simulink model "state_space_all2"  (R2018a)
settings: Solver=FixedStepAuto  StartTime=0.0  StopTime=3  FixedStep=tm  MaxStep=1e-4  RelTol=1e-5  AbsTol=1e-5
InitFcn:
  | SimulinkInit_linea_transmision
values from neighbouring files (symbols this model uses):
  b = 4.91    [SimulinkInit_linea_transmision.m]
  C = 1    [SimulinkInit_linea_transmision.m]
  C1 = 22e-6    (= 2.2e-05)    [SimulinkInit_linea_transmision.m]
  C2 = 22e-6    (= 2.2e-05)    [SimulinkInit_linea_transmision.m]
  C3 = 610e-6    (= 0.00061)    [SimulinkInit_linea_transmision.m]
  Cl = 20000e-6    (= 0.02)    [SimulinkInit_linea_transmision.m]
  Jd = 0.3    [SimulinkInit_linea_transmision.m]
  K = 25    [SimulinkInit_linea_transmision.m]    (also in uio_linear.m = K1+E*H)
  K1 = 9.66    [SimulinkInit_linea_transmision.m]    (also in uio_linear.m = K1')
  K11 = 0.8    [SimulinkInit_linea_transmision.m]
  K1d = 1.15    [SimulinkInit_linea_transmision.m]
  K2 = 6.97    [SimulinkInit_linea_transmision.m]
  K22 = 0.2    [SimulinkInit_linea_transmision.m]
  K2d = 1    [SimulinkInit_linea_transmision.m]
  K3 = 31.8    [SimulinkInit_linea_transmision.m]
  K33 = 0.23    [SimulinkInit_linea_transmision.m]
  K3d = 1    [SimulinkInit_linea_transmision.m]
  K4 = 15.1    [SimulinkInit_linea_transmision.m]
  Kd = 0.02    [SimulinkInit_linea_transmision.m]
  Kdc = 0.02    [SimulinkInit_linea_transmision.m]
  Kf = 1    [SimulinkInit_linea_transmision.m]
  Kh = 1.2    [SimulinkInit_linea_transmision.m]
  Ks = 21.5    [SimulinkInit_linea_transmision.m]
  Ksc = 3    [SimulinkInit_linea_transmision.m]
  Kv = 1    [SimulinkInit_linea_transmision.m]
  L = 5.2    [SimulinkInit_linea_transmision.m]
  L1 = 40e-3    (= 0.04)    [SimulinkInit_linea_transmision.m]
  L2 = 30e-3    (= 0.03)    [SimulinkInit_linea_transmision.m]
  L3 = 5e-3    (= 0.005)    [SimulinkInit_linea_transmision.m]
  L4 = 35e-6    (= 3.5e-05)    [SimulinkInit_linea_transmision.m]
  L5 = 22e-6    (= 2.2e-05)    [SimulinkInit_linea_transmision.m]
  L6 = 10e-6    (= 1e-05)    [SimulinkInit_linea_transmision.m]
  Pd = 0.1    [SimulinkInit_linea_transmision.m]
  R = 10    [SimulinkInit_linea_transmision.m]
  R1 = 0.1    [SimulinkInit_linea_transmision.m]
  R2 = 0.2    [SimulinkInit_linea_transmision.m]
  R3 = 1e-3    (= 0.001)    [SimulinkInit_linea_transmision.m]
  R4 = 0.005    [SimulinkInit_linea_transmision.m]
  R5 = 0.0012    [SimulinkInit_linea_transmision.m]
  R6 = 0.001    [SimulinkInit_linea_transmision.m]
  RL = 10    [SimulinkInit_linea_transmision.m]
  Sbin = 13.8    [SimulinkInit_linea_transmision.m]
  Svin = 2.91    [SimulinkInit_linea_transmision.m]
  T1 = 0.4    [SimulinkInit_linea_transmision.m]
  T2 = 1    [SimulinkInit_linea_transmision.m]
  T3 = 15    [SimulinkInit_linea_transmision.m]
  T4 = 2.5    [SimulinkInit_linea_transmision.m]
  Tao1d = 0.5    [SimulinkInit_linea_transmision.m]
  Tao2d = 0.125    [SimulinkInit_linea_transmision.m]
  Tcd = 0.2    [SimulinkInit_linea_transmision.m]
  Tcr = 0.01    [SimulinkInit_linea_transmision.m]
  Tf = 0.04    [SimulinkInit_linea_transmision.m]
  Tr = 950    [SimulinkInit_linea_transmision.m]
  Tt = 450    [SimulinkInit_linea_transmision.m]
  Ttd = 0.04    [SimulinkInit_linea_transmision.m]
  Tv = 0.05    [SimulinkInit_linea_transmision.m]
  V = 20    [SimulinkInit_linea_transmision.m]
  wref = 70000    [SimulinkInit_linea_transmision.m]
  X_acid = 1.2    [SimulinkInit_linea_transmision.m]
  X_meth = 0.35    [SimulinkInit_linea_transmision.m]
  Z = 3    [SimulinkInit_linea_transmision.m]
undefined symbols (not defined in the file or in its folder): Ad, ataque, Bd, c11, c12, c13, c14, C1o, c21, c22, c23, c24, C2o, c31, c32, c33, c34, C3o, c41, c42, c43, c44, C4o, Cd, F1, F2, F3, F4, H1, H2, H3, H4, K1U, K2U, K3U, K4U, T1s, T2s, T3s, T4s, T5s, tao1, tao2, taod, tm
libraries: neural x277, dsparch4 x4, powerlib_meascontrol x4, mpclib x1, simulink x1
(part 2 of 15)

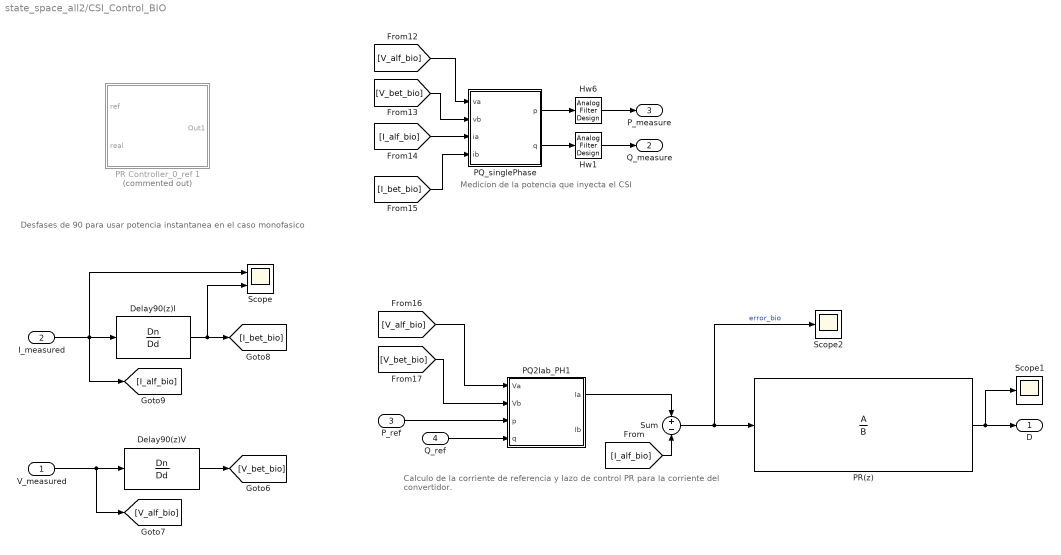
== system state_space_all2/CSI_Control_BIO ==
  note: Medicion de la potencia que inyecta el CSI
  note: Desfases de 90 para usar potencia
      | instantanea en el caso monofasico
  note: Calculo de la corriente de referencia
      | y lazo de control PR para la corriente
      | del convertidor.
  V_measured : Inport
  I_measured : Inport  Port=2
  P_ref : Inport  Port=3
  Q_ref : Inport  Port=4
  Delay90(z)I : DiscreteTransferFcn  Numerator=Dn  Denominator=Dd  SampleTime=T
  Delay90(z)V : DiscreteTransferFcn  Numerator=Dn  Denominator=Dd  SampleTime=T
  Hw1 : dsparch4/Analog Filter Design  method=Bessel  filttype=Lowpass  N=4  Wlo=30*2*pi  Whi=80  Rp=2  Rs=80
  Hw6 : dsparch4/Analog Filter Design  method=Bessel  filttype=Lowpass  N=4  Wlo=30*2*pi  Whi=80  Rp=2  Rs=80
  PQ2Iab_PH1 : MATLAB Function  TreatAsAtomicUnit=on
  PQ_singlePhase : MATLAB Function  TreatAsAtomicUnit=on
  PR Controller_0_ref 1 : Subsystem  Commented=on  mask{Kp=40/100, Ki=200, wa=2, w0=60*2*pi, st_time=1e-3}
      mask prompts: Kp "Ganancia Proporcional"; Ki "Ganancia Integral"; wa "Ancho camapana resonancia"; w0 "Frecuencia Central"; st_time "Tiempo muerto (Start)"
      mask Display:
      | port_label('input',1,'ref')
      | port_label('input',2,'sens')
      | port_label('output',1,'out')
      | 
      | plot(.4+[0:.01:pi/10], .32+sin(40*[0:.01:pi/10])/13)
      | 
      | plot([.4 .6],.05+[.5 .7])
      | plot([.4 .6],.05+[.9 .7])
      | plot([.4 .4],.05+[.9 .5])
      | 
      | text(.27,.37,'\fontsize{25} \int', 'texmode', 'on')
  PR(z) : DiscreteTransferFcn  Numerator=A  Denominator=B  SampleTime=T
  Scope : Scope  NumInputPorts=2
  Scope1 : Scope
  Scope2 : Scope
  Sum : Sum  Inputs=+-
  D : Outport
  Q_measure : Outport  Port=2
  P_measure : Outport  Port=3
  wires:
  I_measured/1 -> Scope/1, Delay90(z)I/1, [I_alf_bio]
  [V_bet_bio] -> PQ2Iab_PH1/2(Vb)
  Delay90(z)I/1 -> Scope/2, [I_bet_bio]
  [I_bet_bio] -> PQ_singlePhase/4(ib)
  [I_alf_bio] -> PQ_singlePhase/3(ia)
  [V_alf_bio] -> PQ2Iab_PH1/1(Va)
  Delay90(z)V/1 -> [V_bet_bio]
  [V_bet_bio] -> PQ_singlePhase/2(vb)
  [V_alf_bio] -> PQ_singlePhase/1(va)
  V_measured/1 -> Delay90(z)V/1, [V_alf_bio]
  P_ref/1 -> PQ2Iab_PH1/3(p)
  Q_ref/1 -> PQ2Iab_PH1/4(q)
  Sum/1 -> Scope2/1, PR(z)/1  "error_bio"
  [I_alf_bio] -> Sum/2
  PQ2Iab_PH1/1(Ia) -> Sum/1
  PR(z)/1 -> Scope1/1, D/1
  PQ_singlePhase/2(q) -> Hw1/1
  Hw1/1 -> Q_measure/1
  PQ_singlePhase/1(p) -> Hw6/1
  Hw6/1 -> P_measure/1

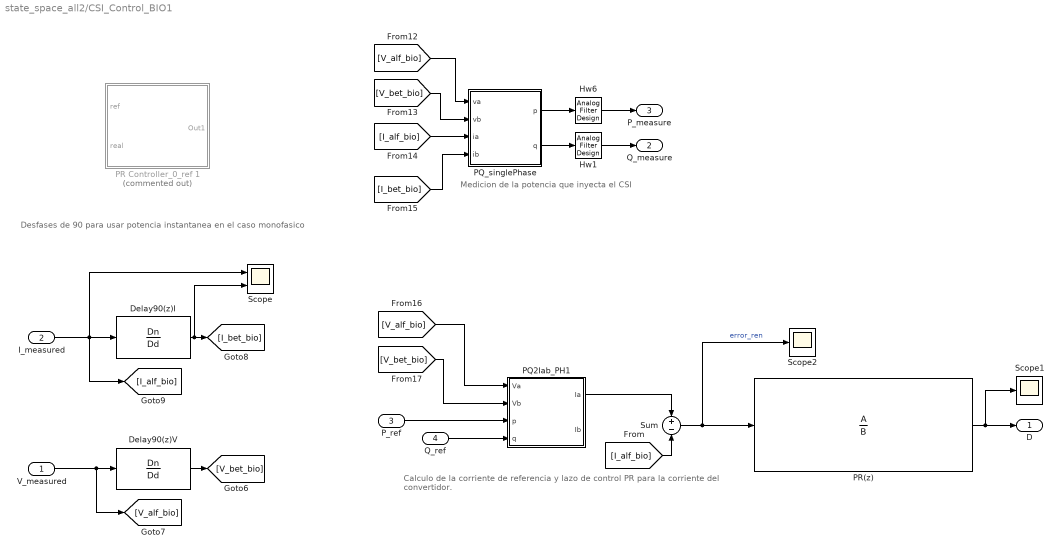
== system state_space_all2/CSI_Control_BIO1 ==
  note: Medicion de la potencia que inyecta el CSI
  note: Desfases de 90 para usar potencia
      | instantanea en el caso monofasico
  note: Calculo de la corriente de referencia
      | y lazo de control PR para la corriente
      | del convertidor.
  V_measured : Inport
  I_measured : Inport  Port=2
  P_ref : Inport  Port=3
  Q_ref : Inport  Port=4
  Delay90(z)I : DiscreteTransferFcn  Numerator=Dn  Denominator=Dd  SampleTime=T
  Delay90(z)V : DiscreteTransferFcn  Numerator=Dn  Denominator=Dd  SampleTime=T
  Hw1 : dsparch4/Analog Filter Design  method=Bessel  filttype=Lowpass  N=4  Wlo=30*2*pi  Whi=80  Rp=2  Rs=80
  Hw6 : dsparch4/Analog Filter Design  method=Bessel  filttype=Lowpass  N=4  Wlo=30*2*pi  Whi=80  Rp=2  Rs=80
  PQ2Iab_PH1 : MATLAB Function  TreatAsAtomicUnit=on
  PQ_singlePhase : MATLAB Function  TreatAsAtomicUnit=on
  PR Controller_0_ref 1 : Subsystem  Commented=on  mask{Kp=40/100, Ki=200, wa=2, w0=60*2*pi, st_time=1e-3}
      mask prompts: Kp "Ganancia Proporcional"; Ki "Ganancia Integral"; wa "Ancho camapana resonancia"; w0 "Frecuencia Central"; st_time "Tiempo muerto (Start)"
      mask Display:
      | port_label('input',1,'ref')
      | port_label('input',2,'sens')
      | port_label('output',1,'out')
      | 
      | plot(.4+[0:.01:pi/10], .32+sin(40*[0:.01:pi/10])/13)
      | 
      | plot([.4 .6],.05+[.5 .7])
      | plot([.4 .6],.05+[.9 .7])
      | plot([.4 .4],.05+[.9 .5])
      | 
      | text(.27,.37,'\fontsize{25} \int', 'texmode', 'on')
  PR(z) : DiscreteTransferFcn  Numerator=A  Denominator=B  SampleTime=T
  Scope : Scope  NumInputPorts=2
  Scope1 : Scope
  Scope2 : Scope
  Sum : Sum  Inputs=+-
  D : Outport
  Q_measure : Outport  Port=2
  P_measure : Outport  Port=3
  wires:
  I_measured/1 -> Scope/1, Delay90(z)I/1, [I_alf_bio]
  [V_bet_bio] -> PQ2Iab_PH1/2(Vb)
  Delay90(z)I/1 -> Scope/2, [I_bet_bio]
  [I_bet_bio] -> PQ_singlePhase/4(ib)
  [I_alf_bio] -> PQ_singlePhase/3(ia)
  [V_alf_bio] -> PQ2Iab_PH1/1(Va)
  Delay90(z)V/1 -> [V_bet_bio]
  [V_bet_bio] -> PQ_singlePhase/2(vb)
  [V_alf_bio] -> PQ_singlePhase/1(va)
  V_measured/1 -> Delay90(z)V/1, [V_alf_bio]
  P_ref/1 -> PQ2Iab_PH1/3(p)
  Q_ref/1 -> PQ2Iab_PH1/4(q)
  Sum/1 -> Scope2/1, PR(z)/1  "error_ren"
  [I_alf_bio] -> Sum/2
  PQ2Iab_PH1/1(Ia) -> Sum/1
  PR(z)/1 -> Scope1/1, D/1
  PQ_singlePhase/2(q) -> Hw1/1
  Hw1/1 -> Q_measure/1
  PQ_singlePhase/1(p) -> Hw6/1
  Hw6/1 -> P_measure/1

== system state_space_all2/Control PR VSI1 ==
  Ierror : Inport
  Constant2 : Constant  Value=0
  Gain2 : Gain  Gain=.002
  Sum5 : Sum  Inputs=+|+
  Sum9 : Sum  Inputs=|++
  Transfer Fcn2 : TransferFcn  Numerator=[2 0]  Denominator=[1 2 (2*pi*60)^2]
  d : Outport
  wires:
  Constant2/1 -> Sum9/2
  Sum5/1 -> Sum9/1
  Transfer Fcn2/1 -> Sum5/2
  Gain2/1 -> Sum5/1
  Ierror/1 -> Transfer Fcn2/1, Gain2/1
  Sum9/1 -> d/1

== system state_space_all2/Diesel Generator2 ==
  in : Inport
  Par de Carga : Inport  Port=2
  " 1" : Gain  Gain=K1d
  " Generador1" : Gain  Gain=1/2
  Actuador1 : TransferFcn  Numerator=[K3d*K2d]  Denominator=[Tao2d 1]
  Dinámica en el eje1 : TransferFcn  Numerator=[(Jd*Pd)]  Denominator=[1 (Jd*Pd)]
  Gain1 : Gain  Gain=12000
  Motor de Combustión1 : TransportDelay  DelayTime=Tao1d
  Sum2 : Sum  Inputs=|+-
  Speed : Outport
  Power : Outport  Port=2
  caudal : Outport  Port=3
  wires:
  " 1"/1 -> Motor de Combustión1/1
  " Generador1"/1 -> Gain1/1
  Motor de Combustión1/1 -> Sum2/1
  Actuador1/1 -> caudal/1, " 1"/1
  Dinámica en el eje1/1 -> Speed/1, " Generador1"/1  "Velocidad"
  Sum2/1 -> Dinámica en el eje1/1
  in/1 -> Actuador1/1
  Par de Carga/1 -> Sum2/2
  Gain1/1 -> Power/1

== system state_space_all2/Function Fitting Neural Network ==
  Input : Inport  PortDimensions=47
      mask Display: e = 0.06;c1 = [120 230 180]/255;c2 = ([120 230 180]+0)/(256+128);c3 = ([120 230 180]+128)/(256+128);patch([0 1 1 0],[0 0 1 1],c1);patch([0 1 1 1-e 1-e 0+e],[0 0 1 1-e 0+e 0+e],c2);patch([0 0 1 1-e 0+e 0+e],[0 1 1 1-e 1-e 0+e],c3);plot([0 1 1 0 0],[0 0 1 1 0]);
  Layer 1 : Subsystem
      mask Display: e = 0.06;c1 = [120 150 230]/255;c2 = ([120 150 230]+0)/383;c3 = ([120 150 230]+128)/383;patch([0 1 1 0],[0 0 1 1],c1);patch([0 1 1 1-e 1-e 0+e],[0 0 1 1-e 0+e 0+e],c2);patch([0 0 1 1-e 0+e 0+e],[0 1 1 1-e 1-e 0+e],c3);plot([0 1 1 0 0],[0 0 1 1 0]);
  Layer 2 : Subsystem
      mask Display: e = 0.06;c1 = [120 150 230]/255;c2 = ([120 150 230]+0)/383;c3 = ([120 150 230]+128)/383;patch([0 1 1 0],[0 0 1 1],c1);patch([0 1 1 1-e 1-e 0+e],[0 0 1 1-e 0+e 0+e],c2);patch([0 0 1 1-e 0+e 0+e],[0 1 1 1-e 1-e 0+e],c3);plot([0 1 1 0 0],[0 0 1 1 0]);
  Layer 3 : Subsystem
      mask Display: e = 0.06;c1 = [120 150 230]/255;c2 = ([120 150 230]+0)/383;c3 = ([120 150 230]+128)/383;patch([0 1 1 0],[0 0 1 1],c1);patch([0 1 1 1-e 1-e 0+e],[0 0 1 1-e 0+e 0+e],c2);patch([0 0 1 1-e 0+e 0+e],[0 1 1 1-e 1-e 0+e],c3);plot([0 1 1 0 0],[0 0 1 1 0]);
  Process Input 1 : Subsystem
      mask Display: e = 0.06;c1 = [120 150 230]/255;c2 = ([120 150 230]+0)/383;c3 = ([120 150 230]+128)/383;patch([0 1 1 0],[0 0 1 1],c1);patch([0 1 1 1-e 1-e 0+e],[0 0 1 1-e 0+e 0+e],c2);patch([0 0 1 1-e 0+e 0+e],[0 1 1 1-e 1-e 0+e],c3);plot([0 1 1 0 0],[0 0 1 1 0]);
  Process Output 1 : Subsystem
      mask Display: e = 0.06;c1 = [120 150 230]/255;c2 = ([120 150 230]+0)/383;c3 = ([120 150 230]+128)/383;patch([0 1 1 0],[0 0 1 1],c1);patch([0 1 1 1-e 1-e 0+e],[0 0 1 1-e 0+e 0+e],c2);patch([0 0 1 1-e 0+e 0+e],[0 1 1 1-e 1-e 0+e],c3);plot([0 1 1 0 0],[0 0 1 1 0]);
  Output : Outport  InitialOutput=[0;0;0;0]
      mask Display: e = 0.06;c1 = [120 230 180]/255;c2 = ([120 230 180]+0)/(256+128);c3 = ([120 230 180]+128)/(256+128);patch([0 1 1 0],[0 0 1 1],c1);patch([0 1 1 1-e 1-e 0+e],[0 0 1 1-e 0+e 0+e],c2);patch([0 0 1 1-e 0+e 0+e],[0 1 1 1-e 1-e 0+e],c3);plot([0 1 1 0 0],[0 0 1 1 0]);
  wires:
  Input/1 -> Process Input 1/1(x)
  Process Output 1/1(y) -> Output/1
  Process Input 1/1(p) -> Layer 1/1("p{1}")
  Layer 1/1("a{1}") -> [feedback1]
  [feedback1] -> Layer 2/1("a{1} ")
  Layer 2/1("a{2}") -> [feedback2]
  [feedback2] -> Layer 3/1("a{2} ")
  Layer 3/1("a{3}") -> Process Output 1/1(a)

== system state_space_all2/Function Fitting Neural Network1 ==
  Input : Inport  PortDimensions=44  SampleTime=4e-05
      mask Display: e = 0.06;c1 = [120 230 180]/255;c2 = ([120 230 180]+0)/(256+128);c3 = ([120 230 180]+128)/(256+128);patch([0 1 1 0],[0 0 1 1],c1);patch([0 1 1 1-e 1-e 0+e],[0 0 1 1-e 0+e 0+e],c2);patch([0 0 1 1-e 0+e 0+e],[0 1 1 1-e 1-e 0+e],c3);plot([0 1 1 0 0],[0 0 1 1 0]);
  Layer 1 : Subsystem
      mask Display: e = 0.06;c1 = [120 150 230]/255;c2 = ([120 150 230]+0)/383;c3 = ([120 150 230]+128)/383;patch([0 1 1 0],[0 0 1 1],c1);patch([0 1 1 1-e 1-e 0+e],[0 0 1 1-e 0+e 0+e],c2);patch([0 0 1 1-e 0+e 0+e],[0 1 1 1-e 1-e 0+e],c3);plot([0 1 1 0 0],[0 0 1 1 0]);
  Layer 2 : Subsystem
      mask Display: e = 0.06;c1 = [120 150 230]/255;c2 = ([120 150 230]+0)/383;c3 = ([120 150 230]+128)/383;patch([0 1 1 0],[0 0 1 1],c1);patch([0 1 1 1-e 1-e 0+e],[0 0 1 1-e 0+e 0+e],c2);patch([0 0 1 1-e 0+e 0+e],[0 1 1 1-e 1-e 0+e],c3);plot([0 1 1 0 0],[0 0 1 1 0]);
  Layer 3 : Subsystem
      mask Display: e = 0.06;c1 = [120 150 230]/255;c2 = ([120 150 230]+0)/383;c3 = ([120 150 230]+128)/383;patch([0 1 1 0],[0 0 1 1],c1);patch([0 1 1 1-e 1-e 0+e],[0 0 1 1-e 0+e 0+e],c2);patch([0 0 1 1-e 0+e 0+e],[0 1 1 1-e 1-e 0+e],c3);plot([0 1 1 0 0],[0 0 1 1 0]);
  Layer 4 : Subsystem
      mask Display: e = 0.06;c1 = [120 150 230]/255;c2 = ([120 150 230]+0)/383;c3 = ([120 150 230]+128)/383;patch([0 1 1 0],[0 0 1 1],c1);patch([0 1 1 1-e 1-e 0+e],[0 0 1 1-e 0+e 0+e],c2);patch([0 0 1 1-e 0+e 0+e],[0 1 1 1-e 1-e 0+e],c3);plot([0 1 1 0 0],[0 0 1 1 0]);
  Process Input 1 : Subsystem
      mask Display: e = 0.06;c1 = [120 150 230]/255;c2 = ([120 150 230]+0)/383;c3 = ([120 150 230]+128)/383;patch([0 1 1 0],[0 0 1 1],c1);patch([0 1 1 1-e 1-e 0+e],[0 0 1 1-e 0+e 0+e],c2);patch([0 0 1 1-e 0+e 0+e],[0 1 1 1-e 1-e 0+e],c3);plot([0 1 1 0 0],[0 0 1 1 0]);
  Process Output 1 : Subsystem
      mask Display: e = 0.06;c1 = [120 150 230]/255;c2 = ([120 150 230]+0)/383;c3 = ([120 150 230]+128)/383;patch([0 1 1 0],[0 0 1 1],c1);patch([0 1 1 1-e 1-e 0+e],[0 0 1 1-e 0+e 0+e],c2);patch([0 0 1 1-e 0+e 0+e],[0 1 1 1-e 1-e 0+e],c3);plot([0 1 1 0 0],[0 0 1 1 0]);
  Output : Outport  InitialOutput=0
      mask Display: e = 0.06;c1 = [120 230 180]/255;c2 = ([120 230 180]+0)/(256+128);c3 = ([120 230 180]+128)/(256+128);patch([0 1 1 0],[0 0 1 1],c1);patch([0 1 1 1-e 1-e 0+e],[0 0 1 1-e 0+e 0+e],c2);patch([0 0 1 1-e 0+e 0+e],[0 1 1 1-e 1-e 0+e],c3);plot([0 1 1 0 0],[0 0 1 1 0]);
  wires:
  Input/1 -> Process Input 1/1(x)
  Process Output 1/1(y) -> Output/1
  Process Input 1/1(p) -> Layer 1/1("p{1}")
  Layer 1/1("a{1}") -> [feedback1]
  [feedback1] -> Layer 2/1("a{1} ")
  Layer 2/1("a{2}") -> [feedback2]
  [feedback2] -> Layer 3/1("a{2} ")
  Layer 3/1("a{3}") -> [feedback3]
  [feedback3] -> Layer 4/1("a{3} ")
  Layer 4/1("a{4}") -> Process Output 1/1(a)

== system state_space_all2/Function Fitting Neural Network2 ==
  Input : Inport  PortDimensions=44  SampleTime=4e-05
      mask Display: e = 0.06;c1 = [120 230 180]/255;c2 = ([120 230 180]+0)/(256+128);c3 = ([120 230 180]+128)/(256+128);patch([0 1 1 0],[0 0 1 1],c1);patch([0 1 1 1-e 1-e 0+e],[0 0 1 1-e 0+e 0+e],c2);patch([0 0 1 1-e 0+e 0+e],[0 1 1 1-e 1-e 0+e],c3);plot([0 1 1 0 0],[0 0 1 1 0]);
  Layer 1 : Subsystem
      mask Display: e = 0.06;c1 = [120 150 230]/255;c2 = ([120 150 230]+0)/383;c3 = ([120 150 230]+128)/383;patch([0 1 1 0],[0 0 1 1],c1);patch([0 1 1 1-e 1-e 0+e],[0 0 1 1-e 0+e 0+e],c2);patch([0 0 1 1-e 0+e 0+e],[0 1 1 1-e 1-e 0+e],c3);plot([0 1 1 0 0],[0 0 1 1 0]);
  Layer 2 : Subsystem
      mask Display: e = 0.06;c1 = [120 150 230]/255;c2 = ([120 150 230]+0)/383;c3 = ([120 150 230]+128)/383;patch([0 1 1 0],[0 0 1 1],c1);patch([0 1 1 1-e 1-e 0+e],[0 0 1 1-e 0+e 0+e],c2);patch([0 0 1 1-e 0+e 0+e],[0 1 1 1-e 1-e 0+e],c3);plot([0 1 1 0 0],[0 0 1 1 0]);
  Layer 3 : Subsystem
      mask Display: e = 0.06;c1 = [120 150 230]/255;c2 = ([120 150 230]+0)/383;c3 = ([120 150 230]+128)/383;patch([0 1 1 0],[0 0 1 1],c1);patch([0 1 1 1-e 1-e 0+e],[0 0 1 1-e 0+e 0+e],c2);patch([0 0 1 1-e 0+e 0+e],[0 1 1 1-e 1-e 0+e],c3);plot([0 1 1 0 0],[0 0 1 1 0]);
  Layer 4 : Subsystem
      mask Display: e = 0.06;c1 = [120 150 230]/255;c2 = ([120 150 230]+0)/383;c3 = ([120 150 230]+128)/383;patch([0 1 1 0],[0 0 1 1],c1);patch([0 1 1 1-e 1-e 0+e],[0 0 1 1-e 0+e 0+e],c2);patch([0 0 1 1-e 0+e 0+e],[0 1 1 1-e 1-e 0+e],c3);plot([0 1 1 0 0],[0 0 1 1 0]);
  Process Input 1 : Subsystem
      mask Display: e = 0.06;c1 = [120 150 230]/255;c2 = ([120 150 230]+0)/383;c3 = ([120 150 230]+128)/383;patch([0 1 1 0],[0 0 1 1],c1);patch([0 1 1 1-e 1-e 0+e],[0 0 1 1-e 0+e 0+e],c2);patch([0 0 1 1-e 0+e 0+e],[0 1 1 1-e 1-e 0+e],c3);plot([0 1 1 0 0],[0 0 1 1 0]);
  Process Output 1 : Subsystem
      mask Display: e = 0.06;c1 = [120 150 230]/255;c2 = ([120 150 230]+0)/383;c3 = ([120 150 230]+128)/383;patch([0 1 1 0],[0 0 1 1],c1);patch([0 1 1 1-e 1-e 0+e],[0 0 1 1-e 0+e 0+e],c2);patch([0 0 1 1-e 0+e 0+e],[0 1 1 1-e 1-e 0+e],c3);plot([0 1 1 0 0],[0 0 1 1 0]);
  Output : Outport  InitialOutput=0
      mask Display: e = 0.06;c1 = [120 230 180]/255;c2 = ([120 230 180]+0)/(256+128);c3 = ([120 230 180]+128)/(256+128);patch([0 1 1 0],[0 0 1 1],c1);patch([0 1 1 1-e 1-e 0+e],[0 0 1 1-e 0+e 0+e],c2);patch([0 0 1 1-e 0+e 0+e],[0 1 1 1-e 1-e 0+e],c3);plot([0 1 1 0 0],[0 0 1 1 0]);
  wires:
  Input/1 -> Process Input 1/1(x)
  Process Output 1/1(y) -> Output/1
  Process Input 1/1(p) -> Layer 1/1("p{1}")
  Layer 1/1("a{1}") -> [feedback1]
  [feedback1] -> Layer 2/1("a{1} ")
  Layer 2/1("a{2}") -> [feedback2]
  [feedback2] -> Layer 3/1("a{2} ")
  Layer 3/1("a{3}") -> [feedback3]
  [feedback3] -> Layer 4/1("a{3} ")
  Layer 4/1("a{4}") -> Process Output 1/1(a)

== system state_space_all2/Function Fitting Neural Network3 ==
  Input : Inport  PortDimensions=44  SampleTime=4e-05
      mask Display: e = 0.06;c1 = [120 230 180]/255;c2 = ([120 230 180]+0)/(256+128);c3 = ([120 230 180]+128)/(256+128);patch([0 1 1 0],[0 0 1 1],c1);patch([0 1 1 1-e 1-e 0+e],[0 0 1 1-e 0+e 0+e],c2);patch([0 0 1 1-e 0+e 0+e],[0 1 1 1-e 1-e 0+e],c3);plot([0 1 1 0 0],[0 0 1 1 0]);
  Layer 1 : Subsystem
      mask Display: e = 0.06;c1 = [120 150 230]/255;c2 = ([120 150 230]+0)/383;c3 = ([120 150 230]+128)/383;patch([0 1 1 0],[0 0 1 1],c1);patch([0 1 1 1-e 1-e 0+e],[0 0 1 1-e 0+e 0+e],c2);patch([0 0 1 1-e 0+e 0+e],[0 1 1 1-e 1-e 0+e],c3);plot([0 1 1 0 0],[0 0 1 1 0]);
  Layer 2 : Subsystem
      mask Display: e = 0.06;c1 = [120 150 230]/255;c2 = ([120 150 230]+0)/383;c3 = ([120 150 230]+128)/383;patch([0 1 1 0],[0 0 1 1],c1);patch([0 1 1 1-e 1-e 0+e],[0 0 1 1-e 0+e 0+e],c2);patch([0 0 1 1-e 0+e 0+e],[0 1 1 1-e 1-e 0+e],c3);plot([0 1 1 0 0],[0 0 1 1 0]);
  Layer 3 : Subsystem
      mask Display: e = 0.06;c1 = [120 150 230]/255;c2 = ([120 150 230]+0)/383;c3 = ([120 150 230]+128)/383;patch([0 1 1 0],[0 0 1 1],c1);patch([0 1 1 1-e 1-e 0+e],[0 0 1 1-e 0+e 0+e],c2);patch([0 0 1 1-e 0+e 0+e],[0 1 1 1-e 1-e 0+e],c3);plot([0 1 1 0 0],[0 0 1 1 0]);
  Layer 4 : Subsystem
      mask Display: e = 0.06;c1 = [120 150 230]/255;c2 = ([120 150 230]+0)/383;c3 = ([120 150 230]+128)/383;patch([0 1 1 0],[0 0 1 1],c1);patch([0 1 1 1-e 1-e 0+e],[0 0 1 1-e 0+e 0+e],c2);patch([0 0 1 1-e 0+e 0+e],[0 1 1 1-e 1-e 0+e],c3);plot([0 1 1 0 0],[0 0 1 1 0]);
  Process Input 1 : Subsystem
      mask Display: e = 0.06;c1 = [120 150 230]/255;c2 = ([120 150 230]+0)/383;c3 = ([120 150 230]+128)/383;patch([0 1 1 0],[0 0 1 1],c1);patch([0 1 1 1-e 1-e 0+e],[0 0 1 1-e 0+e 0+e],c2);patch([0 0 1 1-e 0+e 0+e],[0 1 1 1-e 1-e 0+e],c3);plot([0 1 1 0 0],[0 0 1 1 0]);
  Process Output 1 : Subsystem
      mask Display: e = 0.06;c1 = [120 150 230]/255;c2 = ([120 150 230]+0)/383;c3 = ([120 150 230]+128)/383;patch([0 1 1 0],[0 0 1 1],c1);patch([0 1 1 1-e 1-e 0+e],[0 0 1 1-e 0+e 0+e],c2);patch([0 0 1 1-e 0+e 0+e],[0 1 1 1-e 1-e 0+e],c3);plot([0 1 1 0 0],[0 0 1 1 0]);
  Output : Outport  InitialOutput=0
      mask Display: e = 0.06;c1 = [120 230 180]/255;c2 = ([120 230 180]+0)/(256+128);c3 = ([120 230 180]+128)/(256+128);patch([0 1 1 0],[0 0 1 1],c1);patch([0 1 1 1-e 1-e 0+e],[0 0 1 1-e 0+e 0+e],c2);patch([0 0 1 1-e 0+e 0+e],[0 1 1 1-e 1-e 0+e],c3);plot([0 1 1 0 0],[0 0 1 1 0]);
  wires:
  Input/1 -> Process Input 1/1(x)
  Process Output 1/1(y) -> Output/1
  Process Input 1/1(p) -> Layer 1/1("p{1}")
  Layer 1/1("a{1}") -> [feedback1]
  [feedback1] -> Layer 2/1("a{1} ")
  Layer 2/1("a{2}") -> [feedback2]
  [feedback2] -> Layer 3/1("a{2} ")
  Layer 3/1("a{3}") -> [feedback3]
  [feedback3] -> Layer 4/1("a{3} ")
  Layer 4/1("a{4}") -> Process Output 1/1(a)

== system state_space_all2/Function Fitting Neural Network4 ==
  Input : Inport  PortDimensions=44  SampleTime=4e-05
      mask Display: e = 0.06;c1 = [120 230 180]/255;c2 = ([120 230 180]+0)/(256+128);c3 = ([120 230 180]+128)/(256+128);patch([0 1 1 0],[0 0 1 1],c1);patch([0 1 1 1-e 1-e 0+e],[0 0 1 1-e 0+e 0+e],c2);patch([0 0 1 1-e 0+e 0+e],[0 1 1 1-e 1-e 0+e],c3);plot([0 1 1 0 0],[0 0 1 1 0]);
  Layer 1 : Subsystem
      mask Display: e = 0.06;c1 = [120 150 230]/255;c2 = ([120 150 230]+0)/383;c3 = ([120 150 230]+128)/383;patch([0 1 1 0],[0 0 1 1],c1);patch([0 1 1 1-e 1-e 0+e],[0 0 1 1-e 0+e 0+e],c2);patch([0 0 1 1-e 0+e 0+e],[0 1 1 1-e 1-e 0+e],c3);plot([0 1 1 0 0],[0 0 1 1 0]);
  Layer 2 : Subsystem
      mask Display: e = 0.06;c1 = [120 150 230]/255;c2 = ([120 150 230]+0)/383;c3 = ([120 150 230]+128)/383;patch([0 1 1 0],[0 0 1 1],c1);patch([0 1 1 1-e 1-e 0+e],[0 0 1 1-e 0+e 0+e],c2);patch([0 0 1 1-e 0+e 0+e],[0 1 1 1-e 1-e 0+e],c3);plot([0 1 1 0 0],[0 0 1 1 0]);
  Layer 3 : Subsystem
      mask Display: e = 0.06;c1 = [120 150 230]/255;c2 = ([120 150 230]+0)/383;c3 = ([120 150 230]+128)/383;patch([0 1 1 0],[0 0 1 1],c1);patch([0 1 1 1-e 1-e 0+e],[0 0 1 1-e 0+e 0+e],c2);patch([0 0 1 1-e 0+e 0+e],[0 1 1 1-e 1-e 0+e],c3);plot([0 1 1 0 0],[0 0 1 1 0]);
  Layer 4 : Subsystem
      mask Display: e = 0.06;c1 = [120 150 230]/255;c2 = ([120 150 230]+0)/383;c3 = ([120 150 230]+128)/383;patch([0 1 1 0],[0 0 1 1],c1);patch([0 1 1 1-e 1-e 0+e],[0 0 1 1-e 0+e 0+e],c2);patch([0 0 1 1-e 0+e 0+e],[0 1 1 1-e 1-e 0+e],c3);plot([0 1 1 0 0],[0 0 1 1 0]);
  Process Input 1 : Subsystem
      mask Display: e = 0.06;c1 = [120 150 230]/255;c2 = ([120 150 230]+0)/383;c3 = ([120 150 230]+128)/383;patch([0 1 1 0],[0 0 1 1],c1);patch([0 1 1 1-e 1-e 0+e],[0 0 1 1-e 0+e 0+e],c2);patch([0 0 1 1-e 0+e 0+e],[0 1 1 1-e 1-e 0+e],c3);plot([0 1 1 0 0],[0 0 1 1 0]);
  Process Output 1 : Subsystem
      mask Display: e = 0.06;c1 = [120 150 230]/255;c2 = ([120 150 230]+0)/383;c3 = ([120 150 230]+128)/383;patch([0 1 1 0],[0 0 1 1],c1);patch([0 1 1 1-e 1-e 0+e],[0 0 1 1-e 0+e 0+e],c2);patch([0 0 1 1-e 0+e 0+e],[0 1 1 1-e 1-e 0+e],c3);plot([0 1 1 0 0],[0 0 1 1 0]);
  Output : Outport  InitialOutput=0
      mask Display: e = 0.06;c1 = [120 230 180]/255;c2 = ([120 230 180]+0)/(256+128);c3 = ([120 230 180]+128)/(256+128);patch([0 1 1 0],[0 0 1 1],c1);patch([0 1 1 1-e 1-e 0+e],[0 0 1 1-e 0+e 0+e],c2);patch([0 0 1 1-e 0+e 0+e],[0 1 1 1-e 1-e 0+e],c3);plot([0 1 1 0 0],[0 0 1 1 0]);
  wires:
  Input/1 -> Process Input 1/1(x)
  Process Output 1/1(y) -> Output/1
  Process Input 1/1(p) -> Layer 1/1("p{1}")
  Layer 1/1("a{1}") -> [feedback1]
  [feedback1] -> Layer 2/1("a{1} ")
  Layer 2/1("a{2}") -> [feedback2]
  [feedback2] -> Layer 3/1("a{2} ")
  Layer 3/1("a{3}") -> [feedback3]
  [feedback3] -> Layer 4/1("a{3} ")
  Layer 4/1("a{4}") -> Process Output 1/1(a)

== system state_space_all2/MeasureNode_I1 ==
  in : Inport
  in1 : Inport  Port=2
  Clock : Clock
  MATLAB Function : MATLAB Function  TreatAsAtomicUnit=on
  Out : Outport
  Out1 : Outport  Port=2
  wires:
  MATLAB Function/1(y) -> Out/1
  Clock/1 -> MATLAB Function/1(u1)
  in/1 -> MATLAB Function/2(u2)
  MATLAB Function/2(y2) -> Out1/1
  in1/1 -> MATLAB Function/3(u3)

== system state_space_all2/MeasureNode_I2 ==
  in : Inport
  in1 : Inport  Port=2
  Clock : Clock
  Delay : Delay  DelayLength=10
  MATLAB Function : MATLAB Function  TreatAsAtomicUnit=on
  Out : Outport
  Out1 : Outport  Port=2
  wires:
  MATLAB Function/1(y) -> Delay/1, Out/1
  Clock/1 -> MATLAB Function/1(u1)
  in/1 -> MATLAB Function/2(u2)
  MATLAB Function/2(y2) -> Out1/1
  in1/1 -> MATLAB Function/3(u3)
  Delay/1 -> MATLAB Function/4(u4)

== system state_space_all2/MeasureNode_I3 ==
  in : Inport
  in1 : Inport  Port=2
  Clock : Clock
  MATLAB Function : MATLAB Function  TreatAsAtomicUnit=on
  Out : Outport
  Out1 : Outport  Port=2
  wires:
  MATLAB Function/1(y) -> Out/1
  Clock/1 -> MATLAB Function/1(u1)
  in/1 -> MATLAB Function/2(u2)
  MATLAB Function/2(y2) -> Out1/1
  in1/1 -> MATLAB Function/3(u3)

== system state_space_all2/MeasureNode_I4 ==
  in : Inport
  in1 : Inport  Port=2
  Clock : Clock
  MATLAB Function : MATLAB Function  TreatAsAtomicUnit=on
  Out : Outport
  Out1 : Outport  Port=2
  wires:
  MATLAB Function/1(y) -> Out/1
  Clock/1 -> MATLAB Function/1(u1)
  in/1 -> MATLAB Function/2(u2)
  MATLAB Function/2(y2) -> Out1/1
  in1/1 -> MATLAB Function/3(u3)

== system state_space_all2/MeasureNode_I5 ==
  in : Inport
  Clock : Clock
  MATLAB Function : MATLAB Function  TreatAsAtomicUnit=on
  Out : Outport
  Out1 : Outport  Port=2
  wires:
  MATLAB Function/1(y) -> Out/1
  Clock/1 -> MATLAB Function/1(u1)
  in/1 -> MATLAB Function/2(u2)
  MATLAB Function/2(y2) -> Out1/1

== system state_space_all2/Umbral adaptativo1 ==
  const : Inport
  u : Inport  Port=2
  Abs1 : Abs
  Demux : Demux  Outputs=3
  Demux1 : Demux  Outputs=3
  Demux2 : Demux  Outputs=3
  Gain1 : Gain  Gain=4/3
  Mux2 : Mux  Inputs=3
  Mux3 : Mux  Inputs=3
  Sum2 : Sum  Inputs=|++
  Sum3 : Sum  Inputs=3
  Transfer Fcn10 : TransferFcn  Numerator=[taod 0]/2500  Denominator=[tao2 1]
  Transfer Fcn11 : TransferFcn  Denominator=[tao1 1]
  Transfer Fcn12 : TransferFcn  Denominator=[tao1 1]
  Transfer Fcn5 : TransferFcn  Numerator=[taod 0]/500  Denominator=[tao2 1]
  Transfer Fcn8 : TransferFcn  Denominator=[tao1 1]
  Transfer Fcn9 : TransferFcn  Numerator=[taod 0]/500  Denominator=[tao2 1]
  Out1 : Outport
  wires:
  Demux1/2 -> Transfer Fcn11/1
  Sum2/1 -> Demux1/1
  Mux2/1 -> Sum2/1
  Demux1/1 -> Transfer Fcn8/1
  Gain1/1 -> Sum2/2
  Mux3/1 -> Gain1/1
  Transfer Fcn9/1 -> Mux2/2
  Transfer Fcn8/1 -> Sum3/1
  Demux1/3 -> Transfer Fcn12/1
  Transfer Fcn5/1 -> Mux2/1
  Transfer Fcn11/1 -> Sum3/2
  Transfer Fcn12/1 -> Sum3/3
  Transfer Fcn10/1 -> Mux2/3
  Sum3/1 -> Out1/1
  Demux/2 -> Transfer Fcn9/1
  Demux/1 -> Transfer Fcn5/1
  Demux/3 -> Transfer Fcn10/1
  Demux2/1 -> Mux3/1
  Demux2/2 -> Mux3/2
  Demux2/3 -> Mux3/3
  const/1 -> Demux2/1
  u/1 -> Demux/1

== system state_space_all2/Umbral adaptativo10 ==
  const : Inport
  u : Inport  Port=2
  Abs1 : Abs
  Demux : Demux  Outputs=3
  Demux1 : Demux  Outputs=3
  Demux2 : Demux  Outputs=3
  Gain1 : Gain  Gain=4/3
  Mux2 : Mux  Inputs=3
  Mux3 : Mux  Inputs=3
  Sum2 : Sum  Inputs=|++
  Sum3 : Sum  Inputs=3
  Transfer Fcn10 : TransferFcn  Numerator=[taod 0]/2500  Denominator=[tao2 1]
  Transfer Fcn11 : TransferFcn  Denominator=[tao1 1]
  Transfer Fcn12 : TransferFcn  Denominator=[tao1 1]
  Transfer Fcn5 : TransferFcn  Numerator=[taod 0]/500  Denominator=[tao2 1]
  Transfer Fcn8 : TransferFcn  Denominator=[tao1 1]
  Transfer Fcn9 : TransferFcn  Numerator=[taod 0]/500  Denominator=[tao2 1]
  Out1 : Outport
  wires:
  Demux1/2 -> Transfer Fcn11/1
  Sum2/1 -> Demux1/1
  Mux2/1 -> Sum2/1
  Demux1/1 -> Transfer Fcn8/1
  Gain1/1 -> Sum2/2
  Mux3/1 -> Gain1/1
  Transfer Fcn9/1 -> Mux2/2
  Transfer Fcn8/1 -> Sum3/1
  Demux1/3 -> Transfer Fcn12/1
  Transfer Fcn5/1 -> Mux2/1
  Transfer Fcn11/1 -> Sum3/2
  Transfer Fcn12/1 -> Sum3/3
  Transfer Fcn10/1 -> Mux2/3
  Sum3/1 -> Out1/1
  Demux/2 -> Transfer Fcn9/1
  Demux/1 -> Transfer Fcn5/1
  Demux/3 -> Transfer Fcn10/1
  Demux2/1 -> Mux3/1
  Demux2/2 -> Mux3/2
  Demux2/3 -> Mux3/3
  const/1 -> Demux2/1
  u/1 -> Demux/1

== system state_space_all2/Umbral adaptativo11 ==
  const : Inport
  u : Inport  Port=2
  Abs1 : Abs
  Demux : Demux  Outputs=3
  Demux1 : Demux  Outputs=3
  Demux2 : Demux  Outputs=3
  Gain1 : Gain  Gain=4/3
  Mux2 : Mux  Inputs=3
  Mux3 : Mux  Inputs=3
  Sum2 : Sum  Inputs=|++
  Sum3 : Sum  Inputs=3
  Transfer Fcn10 : TransferFcn  Numerator=[taod 0]/2500  Denominator=[tao2 1]
  Transfer Fcn11 : TransferFcn  Denominator=[tao1 1]
  Transfer Fcn12 : TransferFcn  Denominator=[tao1 1]
  Transfer Fcn5 : TransferFcn  Numerator=[taod 0]/500  Denominator=[tao2 1]
  Transfer Fcn8 : TransferFcn  Denominator=[tao1 1]
  Transfer Fcn9 : TransferFcn  Numerator=[taod 0]/500  Denominator=[tao2 1]
  Out1 : Outport
  wires:
  Demux1/2 -> Transfer Fcn11/1
  Sum2/1 -> Demux1/1
  Mux2/1 -> Sum2/1
  Demux1/1 -> Transfer Fcn8/1
  Gain1/1 -> Sum2/2
  Mux3/1 -> Gain1/1
  Transfer Fcn9/1 -> Mux2/2
  Transfer Fcn8/1 -> Sum3/1
  Demux1/3 -> Transfer Fcn12/1
  Transfer Fcn5/1 -> Mux2/1
  Transfer Fcn11/1 -> Sum3/2
  Transfer Fcn12/1 -> Sum3/3
  Transfer Fcn10/1 -> Mux2/3
  Sum3/1 -> Out1/1
  Demux/2 -> Transfer Fcn9/1
  Demux/1 -> Transfer Fcn5/1
  Demux/3 -> Transfer Fcn10/1
  Demux2/1 -> Mux3/1
  Demux2/2 -> Mux3/2
  Demux2/3 -> Mux3/3
  const/1 -> Demux2/1
  u/1 -> Demux/1

== system state_space_all2/Umbral adaptativo12 ==
  const : Inport
  u : Inport  Port=2
  Abs1 : Abs
  Demux : Demux  Outputs=3
  Demux1 : Demux  Outputs=3
  Demux2 : Demux  Outputs=3
  Gain1 : Gain  Gain=4/3
  Mux2 : Mux  Inputs=3
  Mux3 : Mux  Inputs=3
  Sum2 : Sum  Inputs=|++
  Sum3 : Sum  Inputs=3
  Transfer Fcn10 : TransferFcn  Numerator=[taod 0]/2500  Denominator=[tao2 1]
  Transfer Fcn11 : TransferFcn  Denominator=[tao1 1]
  Transfer Fcn12 : TransferFcn  Denominator=[tao1 1]
  Transfer Fcn5 : TransferFcn  Numerator=[taod 0]/500  Denominator=[tao2 1]
  Transfer Fcn8 : TransferFcn  Denominator=[tao1 1]
  Transfer Fcn9 : TransferFcn  Numerator=[taod 0]/500  Denominator=[tao2 1]
  Out1 : Outport
  wires:
  Demux1/2 -> Transfer Fcn11/1
  Sum2/1 -> Demux1/1
  Mux2/1 -> Sum2/1
  Demux1/1 -> Transfer Fcn8/1
  Gain1/1 -> Sum2/2
  Mux3/1 -> Gain1/1
  Transfer Fcn9/1 -> Mux2/2
  Transfer Fcn8/1 -> Sum3/1
  Demux1/3 -> Transfer Fcn12/1
  Transfer Fcn5/1 -> Mux2/1
  Transfer Fcn11/1 -> Sum3/2
  Transfer Fcn12/1 -> Sum3/3
  Transfer Fcn10/1 -> Mux2/3
  Sum3/1 -> Out1/1
  Demux/2 -> Transfer Fcn9/1
  Demux/1 -> Transfer Fcn5/1
  Demux/3 -> Transfer Fcn10/1
  Demux2/1 -> Mux3/1
  Demux2/2 -> Mux3/2
  Demux2/3 -> Mux3/3
  const/1 -> Demux2/1
  u/1 -> Demux/1

== system state_space_all2/Umbral adaptativo13 ==
  const : Inport
  u : Inport  Port=2
  Abs1 : Abs
  Demux : Demux  Outputs=3
  Demux1 : Demux  Outputs=3
  Demux2 : Demux  Outputs=3
  Gain1 : Gain  Gain=4/3
  Mux2 : Mux  Inputs=3
  Mux3 : Mux  Inputs=3
  Sum2 : Sum  Inputs=|++
  Sum3 : Sum  Inputs=3
  Transfer Fcn10 : TransferFcn  Numerator=[taod 0]/2500  Denominator=[tao2 1]
  Transfer Fcn11 : TransferFcn  Denominator=[tao1 1]
  Transfer Fcn12 : TransferFcn  Denominator=[tao1 1]
  Transfer Fcn5 : TransferFcn  Numerator=[taod 0]/500  Denominator=[tao2 1]
  Transfer Fcn8 : TransferFcn  Denominator=[tao1 1]
  Transfer Fcn9 : TransferFcn  Numerator=[taod 0]/500  Denominator=[tao2 1]
  Out1 : Outport
  wires:
  Demux1/2 -> Transfer Fcn11/1
  Sum2/1 -> Demux1/1
  Mux2/1 -> Sum2/1
  Demux1/1 -> Transfer Fcn8/1
  Gain1/1 -> Sum2/2
  Mux3/1 -> Gain1/1
  Transfer Fcn9/1 -> Mux2/2
  Transfer Fcn8/1 -> Sum3/1
  Demux1/3 -> Transfer Fcn12/1
  Transfer Fcn5/1 -> Mux2/1
  Transfer Fcn11/1 -> Sum3/2
  Transfer Fcn12/1 -> Sum3/3
  Transfer Fcn10/1 -> Mux2/3
  Sum3/1 -> Out1/1
  Demux/2 -> Transfer Fcn9/1
  Demux/1 -> Transfer Fcn5/1
  Demux/3 -> Transfer Fcn10/1
  Demux2/1 -> Mux3/1
  Demux2/2 -> Mux3/2
  Demux2/3 -> Mux3/3
  const/1 -> Demux2/1
  u/1 -> Demux/1

== system state_space_all2/Umbral adaptativo14 ==
  const : Inport
  u : Inport  Port=2
  Abs1 : Abs
  Demux : Demux  Outputs=3
  Demux1 : Demux  Outputs=3
  Demux2 : Demux  Outputs=3
  Gain1 : Gain  Gain=4/3
  Mux2 : Mux  Inputs=3
  Mux3 : Mux  Inputs=3
  Sum2 : Sum  Inputs=|++
  Sum3 : Sum  Inputs=3
  Transfer Fcn10 : TransferFcn  Numerator=[taod 0]/2500  Denominator=[tao2 1]
  Transfer Fcn11 : TransferFcn  Denominator=[tao1 1]
  Transfer Fcn12 : TransferFcn  Denominator=[tao1 1]
  Transfer Fcn5 : TransferFcn  Numerator=[taod 0]/500  Denominator=[tao2 1]
  Transfer Fcn8 : TransferFcn  Denominator=[tao1 1]
  Transfer Fcn9 : TransferFcn  Numerator=[taod 0]/500  Denominator=[tao2 1]
  Out1 : Outport
  wires:
  Demux1/2 -> Transfer Fcn11/1
  Sum2/1 -> Demux1/1
  Mux2/1 -> Sum2/1
  Demux1/1 -> Transfer Fcn8/1
  Gain1/1 -> Sum2/2
  Mux3/1 -> Gain1/1
  Transfer Fcn9/1 -> Mux2/2
  Transfer Fcn8/1 -> Sum3/1
  Demux1/3 -> Transfer Fcn12/1
  Transfer Fcn5/1 -> Mux2/1
  Transfer Fcn11/1 -> Sum3/2
  Transfer Fcn12/1 -> Sum3/3
  Transfer Fcn10/1 -> Mux2/3
  Sum3/1 -> Out1/1
  Demux/2 -> Transfer Fcn9/1
  Demux/1 -> Transfer Fcn5/1
  Demux/3 -> Transfer Fcn10/1
  Demux2/1 -> Mux3/1
  Demux2/2 -> Mux3/2
  Demux2/3 -> Mux3/3
  const/1 -> Demux2/1
  u/1 -> Demux/1

== system state_space_all2/Umbral adaptativo15 ==
  const : Inport
  u : Inport  Port=2
  Abs1 : Abs
  Demux : Demux  Outputs=3
  Demux1 : Demux  Outputs=3
  Demux2 : Demux  Outputs=3
  Gain1 : Gain  Gain=4/3
  Mux2 : Mux  Inputs=3
  Mux3 : Mux  Inputs=3
  Sum2 : Sum  Inputs=|++
  Sum3 : Sum  Inputs=3
  Transfer Fcn10 : TransferFcn  Numerator=[taod 0]/2500  Denominator=[tao2 1]
  Transfer Fcn11 : TransferFcn  Denominator=[tao1 1]
  Transfer Fcn12 : TransferFcn  Denominator=[tao1 1]
  Transfer Fcn5 : TransferFcn  Numerator=[taod 0]/500  Denominator=[tao2 1]
  Transfer Fcn8 : TransferFcn  Denominator=[tao1 1]
  Transfer Fcn9 : TransferFcn  Numerator=[taod 0]/500  Denominator=[tao2 1]
  Out1 : Outport
  wires:
  Demux1/2 -> Transfer Fcn11/1
  Sum2/1 -> Demux1/1
  Mux2/1 -> Sum2/1
  Demux1/1 -> Transfer Fcn8/1
  Gain1/1 -> Sum2/2
  Mux3/1 -> Gain1/1
  Transfer Fcn9/1 -> Mux2/2
  Transfer Fcn8/1 -> Sum3/1
  Demux1/3 -> Transfer Fcn12/1
  Transfer Fcn5/1 -> Mux2/1
  Transfer Fcn11/1 -> Sum3/2
  Transfer Fcn12/1 -> Sum3/3
  Transfer Fcn10/1 -> Mux2/3
  Sum3/1 -> Out1/1
  Demux/2 -> Transfer Fcn9/1
  Demux/1 -> Transfer Fcn5/1
  Demux/3 -> Transfer Fcn10/1
  Demux2/1 -> Mux3/1
  Demux2/2 -> Mux3/2
  Demux2/3 -> Mux3/3
  const/1 -> Demux2/1
  u/1 -> Demux/1

== system state_space_all2/Umbral adaptativo16 ==
  const : Inport
  u : Inport  Port=2
  Abs1 : Abs
  Demux : Demux  Outputs=3
  Demux1 : Demux  Outputs=3
  Demux2 : Demux  Outputs=3
  Gain1 : Gain  Gain=4/3
  Mux2 : Mux  Inputs=3
  Mux3 : Mux  Inputs=3
  Sum2 : Sum  Inputs=|++
  Sum3 : Sum  Inputs=3
  Transfer Fcn10 : TransferFcn  Numerator=[taod 0]/2500  Denominator=[tao2 1]
  Transfer Fcn11 : TransferFcn  Denominator=[tao1 1]
  Transfer Fcn12 : TransferFcn  Denominator=[tao1 1]
  Transfer Fcn5 : TransferFcn  Numerator=[taod 0]/500  Denominator=[tao2 1]
  Transfer Fcn8 : TransferFcn  Denominator=[tao1 1]
  Transfer Fcn9 : TransferFcn  Numerator=[taod 0]/500  Denominator=[tao2 1]
  Out1 : Outport
  wires:
  Demux1/2 -> Transfer Fcn11/1
  Sum2/1 -> Demux1/1
  Mux2/1 -> Sum2/1
  Demux1/1 -> Transfer Fcn8/1
  Gain1/1 -> Sum2/2
  Mux3/1 -> Gain1/1
  Transfer Fcn9/1 -> Mux2/2
  Transfer Fcn8/1 -> Sum3/1
  Demux1/3 -> Transfer Fcn12/1
  Transfer Fcn5/1 -> Mux2/1
  Transfer Fcn11/1 -> Sum3/2
  Transfer Fcn12/1 -> Sum3/3
  Transfer Fcn10/1 -> Mux2/3
  Sum3/1 -> Out1/1
  Demux/2 -> Transfer Fcn9/1
  Demux/1 -> Transfer Fcn5/1
  Demux/3 -> Transfer Fcn10/1
  Demux2/1 -> Mux3/1
  Demux2/2 -> Mux3/2
  Demux2/3 -> Mux3/3
  const/1 -> Demux2/1
  u/1 -> Demux/1

== system state_space_all2/Umbral adaptativo17 ==
  const : Inport
  u : Inport  Port=2
  Abs1 : Abs
  Demux : Demux
  Demux1 : Demux
  Demux2 : Demux
  Gain1 : Gain  Gain=4/3
  Mux2 : Mux
  Mux3 : Mux
  Sum2 : Sum  Inputs=|++
  Transfer Fcn{1,5,9..10} (4 alike) : TransferFcn  Numerator=[taod 0]  Denominator=[tao2 1]
  Transfer Fcn{2,8,11..12} (4 alike) : TransferFcn  Denominator=[tao1 1]
  th1 : Outport
  th2 : Outport  Port=2
  th3 : Outport  Port=3
  th4 : Outport  Port=4
  wires:
  Demux1/2 -> Transfer Fcn11/1
  Sum2/1 -> Demux1/1
  Mux2/1 -> Abs1/1
  Demux1/1 -> Transfer Fcn8/1
  Gain1/1 -> Sum2/2
  Mux3/1 -> Gain1/1
  Transfer Fcn9/1 -> Mux2/2
  Demux1/3 -> Transfer Fcn12/1
  Transfer Fcn5/1 -> Mux2/1
  Transfer Fcn10/1 -> Mux2/3
  Demux/2 -> Transfer Fcn9/1
  Demux/1 -> Transfer Fcn5/1
  Demux/3 -> Transfer Fcn10/1
  Demux2/1 -> Mux3/1
  Demux2/2 -> Mux3/2
  Demux2/3 -> Mux3/3
  const/1 -> Demux2/1
  u/1 -> Demux/1
  Abs1/1 -> Sum2/1
  Demux/4 -> Transfer Fcn1/1
  Transfer Fcn1/1 -> Mux2/4
  Demux2/4 -> Mux3/4
  Demux1/4 -> Transfer Fcn2/1
  Transfer Fcn8/1 -> th1/1
  Transfer Fcn11/1 -> th2/1
  Transfer Fcn12/1 -> th3/1
  Transfer Fcn2/1 -> th4/1

== system state_space_all2/Umbral adaptativo2 ==
  const : Inport
  u : Inport  Port=2
  Abs1 : Abs
  Demux : Demux  Outputs=3
  Demux1 : Demux  Outputs=3
  Demux2 : Demux  Outputs=3
  Gain1 : Gain  Gain=4/3
  Mux2 : Mux  Inputs=3
  Mux3 : Mux  Inputs=3
  Sum2 : Sum  Inputs=|++
  Sum3 : Sum  Inputs=3
  Transfer Fcn10 : TransferFcn  Numerator=[taod 0]/2500  Denominator=[tao2 1]
  Transfer Fcn11 : TransferFcn  Denominator=[tao1 1]
  Transfer Fcn12 : TransferFcn  Denominator=[tao1 1]
  Transfer Fcn5 : TransferFcn  Numerator=[taod 0]/500  Denominator=[tao2 1]
  Transfer Fcn8 : TransferFcn  Denominator=[tao1 1]
  Transfer Fcn9 : TransferFcn  Numerator=[taod 0]/500  Denominator=[tao2 1]
  Out1 : Outport
  wires:
  Demux1/2 -> Transfer Fcn11/1
  Sum2/1 -> Demux1/1
  Mux2/1 -> Sum2/1
  Demux1/1 -> Transfer Fcn8/1
  Gain1/1 -> Sum2/2
  Mux3/1 -> Gain1/1
  Transfer Fcn9/1 -> Mux2/2
  Transfer Fcn8/1 -> Sum3/1
  Demux1/3 -> Transfer Fcn12/1
  Transfer Fcn5/1 -> Mux2/1
  Transfer Fcn11/1 -> Sum3/2
  Transfer Fcn12/1 -> Sum3/3
  Transfer Fcn10/1 -> Mux2/3
  Sum3/1 -> Out1/1
  Demux/2 -> Transfer Fcn9/1
  Demux/1 -> Transfer Fcn5/1
  Demux/3 -> Transfer Fcn10/1
  Demux2/1 -> Mux3/1
  Demux2/2 -> Mux3/2
  Demux2/3 -> Mux3/3
  const/1 -> Demux2/1
  u/1 -> Demux/1

== system state_space_all2/Umbral adaptativo3 ==
  const : Inport
  u : Inport  Port=2
  Abs1 : Abs
  Demux : Demux  Outputs=3
  Demux1 : Demux  Outputs=3
  Demux2 : Demux  Outputs=3
  Gain1 : Gain  Gain=4/3
  Mux2 : Mux  Inputs=3
  Mux3 : Mux  Inputs=3
  Sum2 : Sum  Inputs=|++
  Sum3 : Sum  Inputs=3
  Transfer Fcn10 : TransferFcn  Numerator=[taod 0]/2500  Denominator=[tao2 1]
  Transfer Fcn11 : TransferFcn  Denominator=[tao1 1]
  Transfer Fcn12 : TransferFcn  Denominator=[tao1 1]
  Transfer Fcn5 : TransferFcn  Numerator=[taod 0]/500  Denominator=[tao2 1]
  Transfer Fcn8 : TransferFcn  Denominator=[tao1 1]
  Transfer Fcn9 : TransferFcn  Numerator=[taod 0]/500  Denominator=[tao2 1]
  Out1 : Outport
  wires:
  Demux1/2 -> Transfer Fcn11/1
  Sum2/1 -> Demux1/1
  Mux2/1 -> Sum2/1
  Demux1/1 -> Transfer Fcn8/1
  Gain1/1 -> Sum2/2
  Mux3/1 -> Gain1/1
  Transfer Fcn9/1 -> Mux2/2
  Transfer Fcn8/1 -> Sum3/1
  Demux1/3 -> Transfer Fcn12/1
  Transfer Fcn5/1 -> Mux2/1
  Transfer Fcn11/1 -> Sum3/2
  Transfer Fcn12/1 -> Sum3/3
  Transfer Fcn10/1 -> Mux2/3
  Sum3/1 -> Out1/1
  Demux/2 -> Transfer Fcn9/1
  Demux/1 -> Transfer Fcn5/1
  Demux/3 -> Transfer Fcn10/1
  Demux2/1 -> Mux3/1
  Demux2/2 -> Mux3/2
  Demux2/3 -> Mux3/3
  const/1 -> Demux2/1
  u/1 -> Demux/1

== system state_space_all2/Umbral adaptativo4 ==
  const : Inport
  u : Inport  Port=2
  Abs1 : Abs
  Demux : Demux  Outputs=3
  Demux1 : Demux  Outputs=3
  Demux2 : Demux  Outputs=3
  Gain1 : Gain  Gain=4/3
  Mux2 : Mux  Inputs=3
  Mux3 : Mux  Inputs=3
  Sum2 : Sum  Inputs=|++
  Sum3 : Sum  Inputs=3
  Transfer Fcn10 : TransferFcn  Numerator=[taod 0]/2500  Denominator=[tao2 1]
  Transfer Fcn11 : TransferFcn  Denominator=[tao1 1]
  Transfer Fcn12 : TransferFcn  Denominator=[tao1 1]
  Transfer Fcn5 : TransferFcn  Numerator=[taod 0]/500  Denominator=[tao2 1]
  Transfer Fcn8 : TransferFcn  Denominator=[tao1 1]
  Transfer Fcn9 : TransferFcn  Numerator=[taod 0]/500  Denominator=[tao2 1]
  Out1 : Outport
  wires:
  Demux1/2 -> Transfer Fcn11/1
  Sum2/1 -> Demux1/1
  Mux2/1 -> Sum2/1
  Demux1/1 -> Transfer Fcn8/1
  Gain1/1 -> Sum2/2
  Mux3/1 -> Gain1/1
  Transfer Fcn9/1 -> Mux2/2
  Transfer Fcn8/1 -> Sum3/1
  Demux1/3 -> Transfer Fcn12/1
  Transfer Fcn5/1 -> Mux2/1
  Transfer Fcn11/1 -> Sum3/2
  Transfer Fcn12/1 -> Sum3/3
  Transfer Fcn10/1 -> Mux2/3
  Sum3/1 -> Out1/1
  Demux/2 -> Transfer Fcn9/1
  Demux/1 -> Transfer Fcn5/1
  Demux/3 -> Transfer Fcn10/1
  Demux2/1 -> Mux3/1
  Demux2/2 -> Mux3/2
  Demux2/3 -> Mux3/3
  const/1 -> Demux2/1
  u/1 -> Demux/1

== system state_space_all2/Umbral adaptativo5 ==
  const : Inport
  u : Inport  Port=2
  Abs1 : Abs
  Demux : Demux  Outputs=3
  Demux1 : Demux  Outputs=3
  Demux2 : Demux  Outputs=3
  Gain1 : Gain  Gain=4/3
  Mux2 : Mux  Inputs=3
  Mux3 : Mux  Inputs=3
  Sum2 : Sum  Inputs=|++
  Sum3 : Sum  Inputs=3
  Transfer Fcn10 : TransferFcn  Numerator=[taod 0]/2500  Denominator=[tao2 1]
  Transfer Fcn11 : TransferFcn  Denominator=[tao1 1]
  Transfer Fcn12 : TransferFcn  Denominator=[tao1 1]
  Transfer Fcn5 : TransferFcn  Numerator=[taod 0]/500  Denominator=[tao2 1]
  Transfer Fcn8 : TransferFcn  Denominator=[tao1 1]
  Transfer Fcn9 : TransferFcn  Numerator=[taod 0]/500  Denominator=[tao2 1]
  Out1 : Outport
  wires:
  Demux1/2 -> Transfer Fcn11/1
  Sum2/1 -> Demux1/1
  Mux2/1 -> Sum2/1
  Demux1/1 -> Transfer Fcn8/1
  Gain1/1 -> Sum2/2
  Mux3/1 -> Gain1/1
  Transfer Fcn9/1 -> Mux2/2
  Transfer Fcn8/1 -> Sum3/1
  Demux1/3 -> Transfer Fcn12/1
  Transfer Fcn5/1 -> Mux2/1
  Transfer Fcn11/1 -> Sum3/2
  Transfer Fcn12/1 -> Sum3/3
  Transfer Fcn10/1 -> Mux2/3
  Sum3/1 -> Out1/1
  Demux/2 -> Transfer Fcn9/1
  Demux/1 -> Transfer Fcn5/1
  Demux/3 -> Transfer Fcn10/1
  Demux2/1 -> Mux3/1
  Demux2/2 -> Mux3/2
  Demux2/3 -> Mux3/3
  const/1 -> Demux2/1
  u/1 -> Demux/1

== system state_space_all2/Umbral adaptativo6 ==
  const : Inport
  u : Inport  Port=2
  Abs1 : Abs
  Demux : Demux  Outputs=3
  Demux1 : Demux  Outputs=3
  Demux2 : Demux  Outputs=3
  Gain1 : Gain  Gain=4/3
  Mux2 : Mux  Inputs=3
  Mux3 : Mux  Inputs=3
  Sum2 : Sum  Inputs=|++
  Sum3 : Sum  Inputs=3
  Transfer Fcn10 : TransferFcn  Numerator=[taod 0]/2500  Denominator=[tao2 1]
  Transfer Fcn11 : TransferFcn  Denominator=[tao1 1]
  Transfer Fcn12 : TransferFcn  Denominator=[tao1 1]
  Transfer Fcn5 : TransferFcn  Numerator=[taod 0]/500  Denominator=[tao2 1]
  Transfer Fcn8 : TransferFcn  Denominator=[tao1 1]
  Transfer Fcn9 : TransferFcn  Numerator=[taod 0]/500  Denominator=[tao2 1]
  Out1 : Outport
  wires:
  Demux1/2 -> Transfer Fcn11/1
  Sum2/1 -> Demux1/1
  Mux2/1 -> Sum2/1
  Demux1/1 -> Transfer Fcn8/1
  Gain1/1 -> Sum2/2
  Mux3/1 -> Gain1/1
  Transfer Fcn9/1 -> Mux2/2
  Transfer Fcn8/1 -> Sum3/1
  Demux1/3 -> Transfer Fcn12/1
  Transfer Fcn5/1 -> Mux2/1
  Transfer Fcn11/1 -> Sum3/2
  Transfer Fcn12/1 -> Sum3/3
  Transfer Fcn10/1 -> Mux2/3
  Sum3/1 -> Out1/1
  Demux/2 -> Transfer Fcn9/1
  Demux/1 -> Transfer Fcn5/1
  Demux/3 -> Transfer Fcn10/1
  Demux2/1 -> Mux3/1
  Demux2/2 -> Mux3/2
  Demux2/3 -> Mux3/3
  const/1 -> Demux2/1
  u/1 -> Demux/1

== system state_space_all2/Umbral adaptativo7 ==
  const : Inport
  u : Inport  Port=2
  Abs1 : Abs
  Demux : Demux  Outputs=3
  Demux1 : Demux  Outputs=3
  Demux2 : Demux  Outputs=3
  Gain1 : Gain  Gain=4/3
  Mux2 : Mux  Inputs=3
  Mux3 : Mux  Inputs=3
  Sum2 : Sum  Inputs=|++
  Sum3 : Sum  Inputs=3
  Transfer Fcn10 : TransferFcn  Numerator=[taod 0]/2500  Denominator=[tao2 1]
  Transfer Fcn11 : TransferFcn  Denominator=[tao1 1]
  Transfer Fcn12 : TransferFcn  Denominator=[tao1 1]
  Transfer Fcn5 : TransferFcn  Numerator=[taod 0]/500  Denominator=[tao2 1]
  Transfer Fcn8 : TransferFcn  Denominator=[tao1 1]
  Transfer Fcn9 : TransferFcn  Numerator=[taod 0]/500  Denominator=[tao2 1]
  Out1 : Outport
  wires:
  Demux1/2 -> Transfer Fcn11/1
  Sum2/1 -> Demux1/1
  Mux2/1 -> Sum2/1
  Demux1/1 -> Transfer Fcn8/1
  Gain1/1 -> Sum2/2
  Mux3/1 -> Gain1/1
  Transfer Fcn9/1 -> Mux2/2
  Transfer Fcn8/1 -> Sum3/1
  Demux1/3 -> Transfer Fcn12/1
  Transfer Fcn5/1 -> Mux2/1
  Transfer Fcn11/1 -> Sum3/2
  Transfer Fcn12/1 -> Sum3/3
  Transfer Fcn10/1 -> Mux2/3
  Sum3/1 -> Out1/1
  Demux/2 -> Transfer Fcn9/1
  Demux/1 -> Transfer Fcn5/1
  Demux/3 -> Transfer Fcn10/1
  Demux2/1 -> Mux3/1
  Demux2/2 -> Mux3/2
  Demux2/3 -> Mux3/3
  const/1 -> Demux2/1
  u/1 -> Demux/1

== system state_space_all2/Umbral adaptativo8 ==
  const : Inport
  u : Inport  Port=2
  Abs1 : Abs
  Demux : Demux  Outputs=3
  Demux1 : Demux  Outputs=3
  Demux2 : Demux  Outputs=3
  Gain1 : Gain  Gain=4/3
  Mux2 : Mux  Inputs=3
  Mux3 : Mux  Inputs=3
  Sum2 : Sum  Inputs=|++
  Sum3 : Sum  Inputs=3
  Transfer Fcn10 : TransferFcn  Numerator=[taod 0]/2500  Denominator=[tao2 1]
  Transfer Fcn11 : TransferFcn  Denominator=[tao1 1]
  Transfer Fcn12 : TransferFcn  Denominator=[tao1 1]
  Transfer Fcn5 : TransferFcn  Numerator=[taod 0]/500  Denominator=[tao2 1]
  Transfer Fcn8 : TransferFcn  Denominator=[tao1 1]
  Transfer Fcn9 : TransferFcn  Numerator=[taod 0]/500  Denominator=[tao2 1]
  Out1 : Outport
  wires:
  Demux1/2 -> Transfer Fcn11/1
  Sum2/1 -> Demux1/1
  Mux2/1 -> Sum2/1
  Demux1/1 -> Transfer Fcn8/1
  Gain1/1 -> Sum2/2
  Mux3/1 -> Gain1/1
  Transfer Fcn9/1 -> Mux2/2
  Transfer Fcn8/1 -> Sum3/1
  Demux1/3 -> Transfer Fcn12/1
  Transfer Fcn5/1 -> Mux2/1
  Transfer Fcn11/1 -> Sum3/2
  Transfer Fcn12/1 -> Sum3/3
  Transfer Fcn10/1 -> Mux2/3
  Sum3/1 -> Out1/1
  Demux/2 -> Transfer Fcn9/1
  Demux/1 -> Transfer Fcn5/1
  Demux/3 -> Transfer Fcn10/1
  Demux2/1 -> Mux3/1
  Demux2/2 -> Mux3/2
  Demux2/3 -> Mux3/3
  const/1 -> Demux2/1
  u/1 -> Demux/1

== system state_space_all2/Umbral adaptativo9 ==
  const : Inport
  u : Inport  Port=2
  Abs1 : Abs
  Demux : Demux  Outputs=3
  Demux1 : Demux  Outputs=3
  Demux2 : Demux  Outputs=3
  Gain1 : Gain  Gain=4/3
  Mux2 : Mux  Inputs=3
  Mux3 : Mux  Inputs=3
  Sum2 : Sum  Inputs=|++
  Sum3 : Sum  Inputs=3
  Transfer Fcn10 : TransferFcn  Numerator=[taod 0]/2500  Denominator=[tao2 1]
  Transfer Fcn11 : TransferFcn  Denominator=[tao1 1]
  Transfer Fcn12 : TransferFcn  Denominator=[tao1 1]
  Transfer Fcn5 : TransferFcn  Numerator=[taod 0]/500  Denominator=[tao2 1]
  Transfer Fcn8 : TransferFcn  Denominator=[tao1 1]
  Transfer Fcn9 : TransferFcn  Numerator=[taod 0]/500  Denominator=[tao2 1]
  Out1 : Outport
  wires:
  Demux1/2 -> Transfer Fcn11/1
  Sum2/1 -> Demux1/1
  Mux2/1 -> Sum2/1
  Demux1/1 -> Transfer Fcn8/1
  Gain1/1 -> Sum2/2
  Mux3/1 -> Gain1/1
  Transfer Fcn9/1 -> Mux2/2
  Transfer Fcn8/1 -> Sum3/1
  Demux1/3 -> Transfer Fcn12/1
  Transfer Fcn5/1 -> Mux2/1
  Transfer Fcn11/1 -> Sum3/2
  Transfer Fcn12/1 -> Sum3/3
  Transfer Fcn10/1 -> Mux2/3
  Sum3/1 -> Out1/1
  Demux/2 -> Transfer Fcn9/1
  Demux/1 -> Transfer Fcn5/1
  Demux/3 -> Transfer Fcn10/1
  Demux2/1 -> Mux3/1
  Demux2/2 -> Mux3/2
  Demux2/3 -> Mux3/3
  const/1 -> Demux2/1
  u/1 -> Demux/1
